simulink library "Filter_With_Tustin"  (R2019b)
settings: Solver=VariableStepAuto  StartTime=0.0  StopTime=10.0  RelTol=1e-3
settings Model: Creator=Edoardo  LastModifiedBy=Edoardo

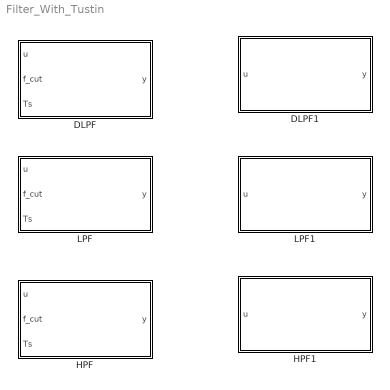
== system Filter_With_Tustin ==
  DLPF : Subsystem
  DLPF1 : Subsystem  mask{f_cut=0, Ts=0}
      mask prompts: f_cut "Cut frequency (Hz)"; Ts "Sampling time (s)"
      mask Display: fprintf('DLPF');
  HPF : Subsystem
  HPF1 : Subsystem  mask{f_cut=0, Ts=0}
      mask prompts: f_cut "Cut frequency (Hz)"; Ts "Sampling time (s)"
      mask Display: fprintf('HPF')
  LPF : Subsystem
  LPF1 : Subsystem  mask{f_cut=0, Ts=0}
      mask prompts: f_cut "Cut frequency (Hz)"; Ts "Sampling time (s)"
      mask Display: fprintf('LPF')

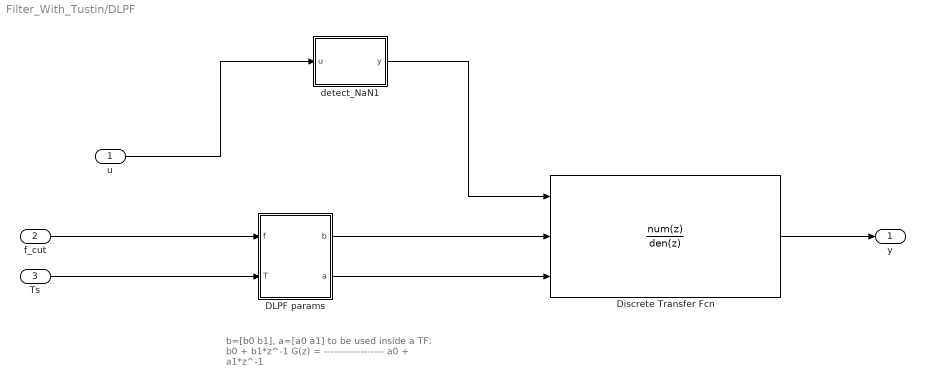
== system Filter_With_Tustin/DLPF ==
  note: b=[b0 b1], a=[a0 a1] to be used inside a TF:
      |                             b0 + b1*z^-1
      |                  G(z) = ------------------
      |                             a0 + a1*z^-1
  u : Inport
  f_cut : Inport  Port=2
  Ts : Inport  Port=3
  "DLPF params " : MATLAB Function  TreatAsAtomicUnit=on
  Discrete Transfer Fcn : DiscreteTransferFcn  NumeratorSource=Input port  DenominatorSource=Input port  a0EqualsOne=on
      settings: InputPortMap=u0,p1,p3
  detect_NaN1 : MATLAB Function  TreatAsAtomicUnit=on
  y : Outport
  wires:
  f_cut/1 -> "DLPF params "/1(f)
  "DLPF params "/2(a) -> Discrete Transfer Fcn/3
  Discrete Transfer Fcn/1 -> y/1
  Ts/1 -> "DLPF params "/2(T)
  "DLPF params "/1(b) -> Discrete Transfer Fcn/2
  u/1 -> detect_NaN1/1(u)
  detect_NaN1/1(y) -> Discrete Transfer Fcn/1

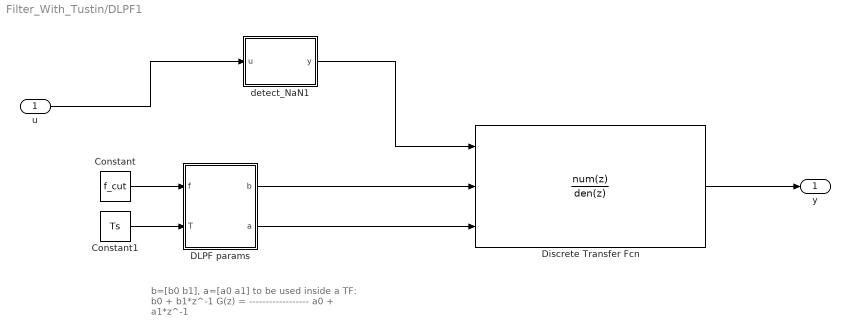
== system Filter_With_Tustin/DLPF1 ==
  note: b=[b0 b1], a=[a0 a1] to be used inside a TF:
      |                             b0 + b1*z^-1
      |                  G(z) = ------------------
      |                             a0 + a1*z^-1
  u : Inport
  Constant : Constant  Value=f_cut
  Constant1 : Constant  Value=Ts
  "DLPF params " : MATLAB Function  TreatAsAtomicUnit=on
  Discrete Transfer Fcn : DiscreteTransferFcn  NumeratorSource=Input port  DenominatorSource=Input port  a0EqualsOne=on
      settings: InputPortMap=u0,p1,p3
  detect_NaN1 : MATLAB Function  TreatAsAtomicUnit=on
  y : Outport
  wires:
  "DLPF params "/1(b) -> Discrete Transfer Fcn/2
  Discrete Transfer Fcn/1 -> y/1
  "DLPF params "/2(a) -> Discrete Transfer Fcn/3
  Constant/1 -> "DLPF params "/1(f)
  Constant1/1 -> "DLPF params "/2(T)
  u/1 -> detect_NaN1/1(u)
  detect_NaN1/1(y) -> Discrete Transfer Fcn/1

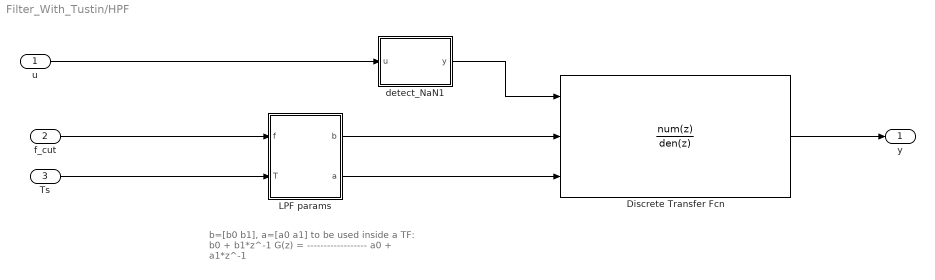
== system Filter_With_Tustin/HPF ==
  note: b=[b0 b1], a=[a0 a1] to be used inside a TF:
      |                             b0 + b1*z^-1
      |                  G(z) = ------------------
      |                             a0 + a1*z^-1
  u : Inport
  f_cut : Inport  Port=2
  Ts : Inport  Port=3
  Discrete Transfer Fcn : DiscreteTransferFcn  NumeratorSource=Input port  DenominatorSource=Input port  a0EqualsOne=on
      settings: InputPortMap=u0,p1,p3
  "LPF params " : MATLAB Function  TreatAsAtomicUnit=on
  detect_NaN1 : MATLAB Function  TreatAsAtomicUnit=on
  y : Outport
  wires:
  f_cut/1 -> "LPF params "/1(f)
  "LPF params "/2(a) -> Discrete Transfer Fcn/3
  Discrete Transfer Fcn/1 -> y/1
  Ts/1 -> "LPF params "/2(T)
  "LPF params "/1(b) -> Discrete Transfer Fcn/2
  u/1 -> detect_NaN1/1(u)
  detect_NaN1/1(y) -> Discrete Transfer Fcn/1

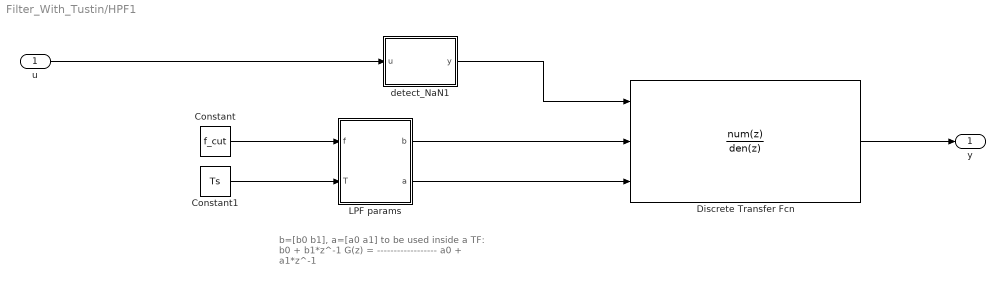
== system Filter_With_Tustin/HPF1 ==
  note: b=[b0 b1], a=[a0 a1] to be used inside a TF:
      |                             b0 + b1*z^-1
      |                  G(z) = ------------------
      |                             a0 + a1*z^-1
  u : Inport
  Constant : Constant  Value=f_cut
  Constant1 : Constant  Value=Ts
  Discrete Transfer Fcn : DiscreteTransferFcn  NumeratorSource=Input port  DenominatorSource=Input port  a0EqualsOne=on
      settings: InputPortMap=u0,p1,p3
  "LPF params " : MATLAB Function  TreatAsAtomicUnit=on
  detect_NaN1 : MATLAB Function  TreatAsAtomicUnit=on
  y : Outport
  wires:
  Constant/1 -> "LPF params "/1(f)
  Constant1/1 -> "LPF params "/2(T)
  "LPF params "/1(b) -> Discrete Transfer Fcn/2
  Discrete Transfer Fcn/1 -> y/1
  "LPF params "/2(a) -> Discrete Transfer Fcn/3
  u/1 -> detect_NaN1/1(u)
  detect_NaN1/1(y) -> Discrete Transfer Fcn/1

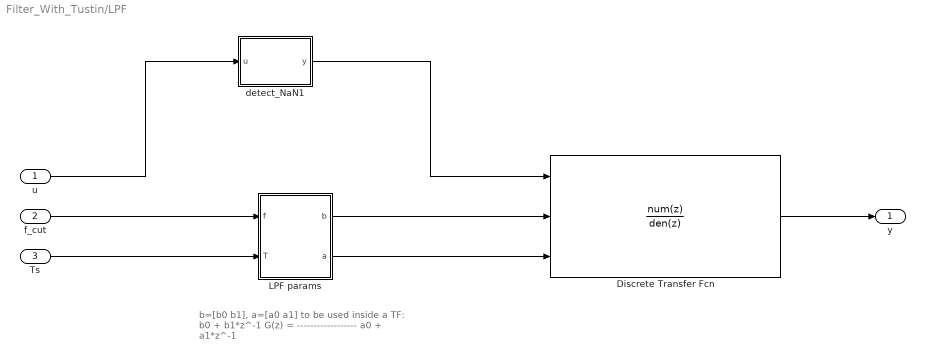
== system Filter_With_Tustin/LPF ==
  note: b=[b0 b1], a=[a0 a1] to be used inside a TF:
      |                             b0 + b1*z^-1
      |                  G(z) = ------------------
      |                             a0 + a1*z^-1
  u : Inport
  f_cut : Inport  Port=2
  Ts : Inport  Port=3
  Discrete Transfer Fcn : DiscreteTransferFcn  NumeratorSource=Input port  DenominatorSource=Input port  a0EqualsOne=on
      settings: InputPortMap=u0,p1,p3
  "LPF params " : MATLAB Function  TreatAsAtomicUnit=on
  detect_NaN1 : MATLAB Function  TreatAsAtomicUnit=on
  y : Outport
  wires:
  "LPF params "/1(b) -> Discrete Transfer Fcn/2
  Ts/1 -> "LPF params "/2(T)
  Discrete Transfer Fcn/1 -> y/1
  "LPF params "/2(a) -> Discrete Transfer Fcn/3
  f_cut/1 -> "LPF params "/1(f)
  u/1 -> detect_NaN1/1(u)
  detect_NaN1/1(y) -> Discrete Transfer Fcn/1

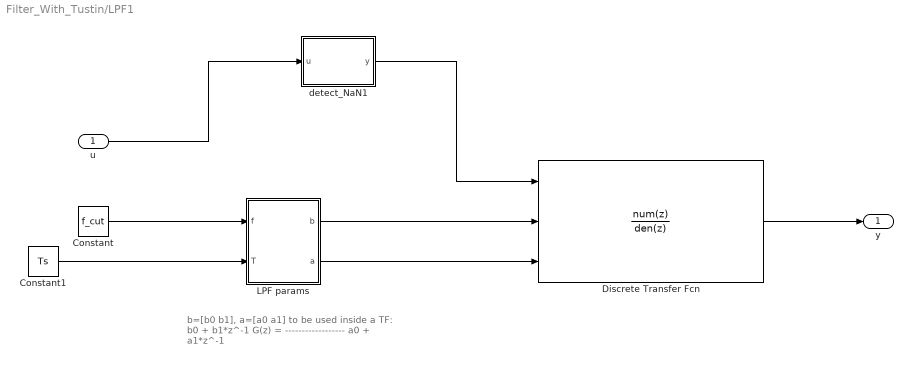
== system Filter_With_Tustin/LPF1 ==
  note: b=[b0 b1], a=[a0 a1] to be used inside a TF:
      |                             b0 + b1*z^-1
      |                  G(z) = ------------------
      |                             a0 + a1*z^-1
  u : Inport
  Constant : Constant  Value=f_cut
  Constant1 : Constant  Value=Ts
  Discrete Transfer Fcn : DiscreteTransferFcn  NumeratorSource=Input port  DenominatorSource=Input port  a0EqualsOne=on
      settings: InputPortMap=u0,p1,p3
  "LPF params " : MATLAB Function  TreatAsAtomicUnit=on
  detect_NaN1 : MATLAB Function  TreatAsAtomicUnit=on
  y : Outport
  wires:
  "LPF params "/2(a) -> Discrete Transfer Fcn/3
  Discrete Transfer Fcn/1 -> y/1
  "LPF params "/1(b) -> Discrete Transfer Fcn/2
  Constant1/1 -> "LPF params "/2(T)
  Constant/1 -> "LPF params "/1(f)
  u/1 -> detect_NaN1/1(u)
  detect_NaN1/1(y) -> Discrete Transfer Fcn/1

== matlab function Filter_With_Tustin/LPF/LPF params  ==
  data: f input; T input; b output; a output
function [b, a] = fcn(f, T)

b0 = pi*f*T/(pi*f*T+1);
b1 = b0;

a0 = 1;
a1 = (pi*f*T-1)/(pi*f*T+1);

a = [a0 a1]; 
b = [b0 b1];

== matlab function Filter_With_Tustin/DLPF1/DLPF params  ==
  data: f input; T input; b output; a output
function [b, a] = fcn(f, T)

b0 = 2*pi*f/(pi*f*T+1);
b1 = -b0;

a0 = 1;
a1 = (pi*f*T-1)/(pi*f*T+1);

b = [b0 b1];
a = [a0 a1];

== matlab function Filter_With_Tustin/LPF1/LPF params  ==
  data: f input; T input; b output; a output
function [b, a] = fcn(f, T)

b0 = pi*f*T/(pi*f*T+1);
b1 = b0;

a0 = 1;
a1 = (pi*f*T-1)/(pi*f*T+1);

a = [a0 a1]; 
b = [b0 b1];

== matlab function Filter_With_Tustin/HPF/LPF params  ==
  data: f input; T input; b output; a output
function [b, a] = fcn(f, T)

b0 = pi*f*T/(pi*f*T+1);
b1 = b0;

a0 = 1;
a1 = (pi*f*T-1)/(pi*f*T+1);

a = [a0 a1]; 
b = [b0 b1];

== matlab function Filter_With_Tustin/HPF1/LPF params  ==
  data: f input; T input; b output; a output
function [b, a] = fcn(f, T)

b0 = pi*f*T/(pi*f*T+1);
b1 = b0;

a0 = 1;
a1 = (pi*f*T-1)/(pi*f*T+1);

a = [a0 a1]; 
b = [b0 b1];

== matlab function Filter_With_Tustin/DLPF/DLPF params  ==
  data: f input; T input; b output; a output
function [b, a] = fcn(f, T)

b0 = 2*pi*f/(pi*f*T+1);
b1 = -b0;

a0 = 1;
a1 = (pi*f*T-1)/(pi*f*T+1);

b = [b0 b1];
a = [a0 a1];

== matlab function Filter_With_Tustin/HPF1/detect_NaN1 ==
  data: u input; y output
function y = detect_NaN(u)
y =u;
 y(isnan(u))= 0;

== matlab function Filter_With_Tustin/LPF1/detect_NaN1 ==
  data: u input; y output
function y = detect_NaN(u)
y =u;
 y(isnan(u))= 0;

== matlab function Filter_With_Tustin/DLPF1/detect_NaN1 ==
  data: u input; y output
function y = detect_NaN(u)
y =u;
 y(isnan(u))= 0;

== matlab function Filter_With_Tustin/DLPF/detect_NaN1 ==
  data: u input; y output
function y = detect_NaN(u)


y =u;
 y(isnan(u))= 0;

== matlab function Filter_With_Tustin/LPF/detect_NaN1 ==
  data: u input; y output
function y = detect_NaN(u)


y =u;
 y(isnan(u))= 0;

== matlab function Filter_With_Tustin/HPF/detect_NaN1 ==
  data: u input; y output
function y = detect_NaN(u)
y =u;
 y(isnan(u))= 0;
